simulink model "lab05_5"  (R2018b)
settings: Solver=VariableStepAuto  StartTime=0.0  StopTime=25  RelTol=1e-3
settings Model: Creator=Ivan  LastModifiedBy=Ivan

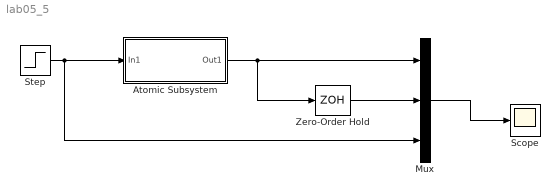
== system lab05_5 ==
  Atomic Subsystem : Subsystem  TreatAsAtomicUnit=on
  Mux : Mux  Inputs=3
  Scope : Scope
  Step : Step  Before=1  SampleTime=0.5
  Zero-Order Hold : ZeroOrderHold  SampleTime=-1
  wires:
  Step/1 -> Mux/3, Atomic Subsystem/1(In1)
  Atomic Subsystem/1(Out1) -> Zero-Order Hold/1, Mux/1
  Zero-Order Hold/1 -> Mux/2
  Mux/1 -> Scope/1

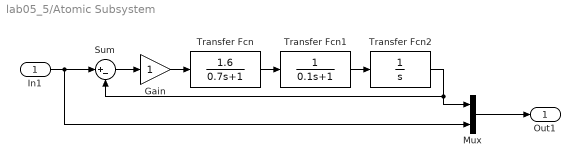
== system lab05_5/Atomic Subsystem ==
  In1 : Inport
  Gain : Gain
  Mux : Mux  Inputs=2
  Sum : Sum  Inputs=|+-
  Transfer Fcn : TransferFcn  Numerator=[1.6]  Denominator=[0.7 1]
  Transfer Fcn1 : TransferFcn  Denominator=[0.1 1]
  Transfer Fcn2 : TransferFcn  Denominator=[1 0]
  Out1 : Outport
  wires:
  Transfer Fcn/1 -> Transfer Fcn1/1
  Mux/1 -> Out1/1
  Transfer Fcn2/1 -> Sum/2, Mux/1
  Transfer Fcn1/1 -> Transfer Fcn2/1
  In1/1 -> Mux/2, Sum/1
  Sum/1 -> Gain/1
  Gain/1 -> Transfer Fcn/1
